simulink model "ss_robust_estimator_CT_real"  (R2022b)
settings: Solver=VariableStepAuto  StartTime=0.0  StopTime=10.0  FixedStep=Ts/20  RelTol=1e-3
undefined symbols (not defined in the file): degs2rpm, der, drv, gbox, mld, mot, rads2rpm, redObs, rpm2rads, sens, simul, ssNominal, ssRobust, Ts
settings Model: Creator=emanuelevitetta  LastModifiedBy=david

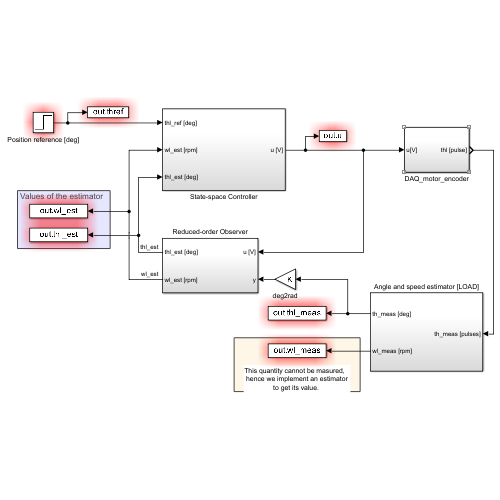
[thumbnail: Simulink's stored preview of the top-level diagram]
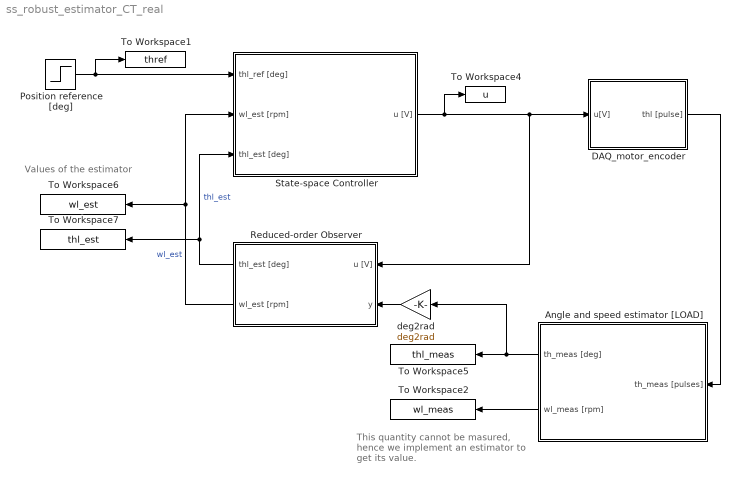
== system ss_robust_estimator_CT_real ==
  note: This quantity cannot be masured,
      | hence we implement an estimator
      | to get its value.
  note: Values of the estimator
  Angle and speed estimator [LOAD] : Subsystem
  DAQ_motor_encoder : Subsystem
  Position reference [deg] : Step  After=simul.stepdeg
  Reduced-order Observer : Subsystem
  State-space Controller : Subsystem
  To Workspace1 : ToWorkspace  VariableName=thref  SaveFormat=Structure With Time  SampleTime=Ts
  To Workspace2 : ToWorkspace  VariableName=wl_meas  SaveFormat=Structure With Time  SampleTime=Ts
  To Workspace4 : ToWorkspace  VariableName=u  SaveFormat=Structure With Time  SampleTime=Ts
  To Workspace5 : ToWorkspace  VariableName=thl_meas  SaveFormat=Structure With Time  SampleTime=Ts
  To Workspace6 : ToWorkspace  VariableName=wl_est  SaveFormat=Structure With Time  SampleTime=Ts
  To Workspace7 : ToWorkspace  VariableName=thl_est  SaveFormat=Structure With Time  SampleTime=Ts
  deg2rad : Gain  Gain=deg2rad
  wires:
  DAQ_motor_encoder/1(thl [pulse]) -> Angle and speed estimator [LOAD]/1(th_meas [pulses])
  Position reference [deg]/1 -> To Workspace1/1, State-space Controller/1(thl_ref [deg])
  Reduced-order Observer/2(wl_est [rpm]) -> To Workspace6/1, State-space Controller/2(wl_est [rpm])  "wl_est"
  State-space Controller/1(u [V]) -> To Workspace4/1, DAQ_motor_encoder/1(u[V]), Reduced-order Observer/1(u [V])
  Reduced-order Observer/1(thl_est [deg]) -> State-space Controller/3(thl_est [deg]), To Workspace7/1  "thl_est"
  deg2rad/1 -> Reduced-order Observer/2(y)
  Angle and speed estimator [LOAD]/1(th_meas [deg]) -> deg2rad/1, To Workspace5/1
  Angle and speed estimator [LOAD]/2(wl_meas [rpm]) -> To Workspace2/1

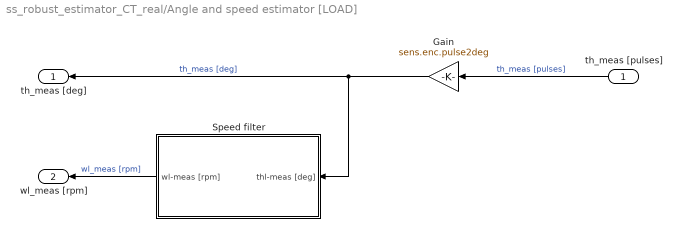
== system ss_robust_estimator_CT_real/Angle and speed estimator [LOAD] ==
  th_meas [pulses] : Inport
  Gain : Gain  Gain=sens.enc.pulse2deg
  Speed filter : Subsystem
  th_meas [deg] : Outport
  wl_meas [rpm] : Outport  Port=2
  wires:
  Speed filter/1(wl-meas [rpm]) -> wl_meas [rpm]/1  "wl_meas [rpm]"
  th_meas [pulses]/1 -> Gain/1  "th_meas [pulses]"
  Gain/1 -> Speed filter/1(thl-meas [deg]), th_meas [deg]/1  "th_meas [deg]"

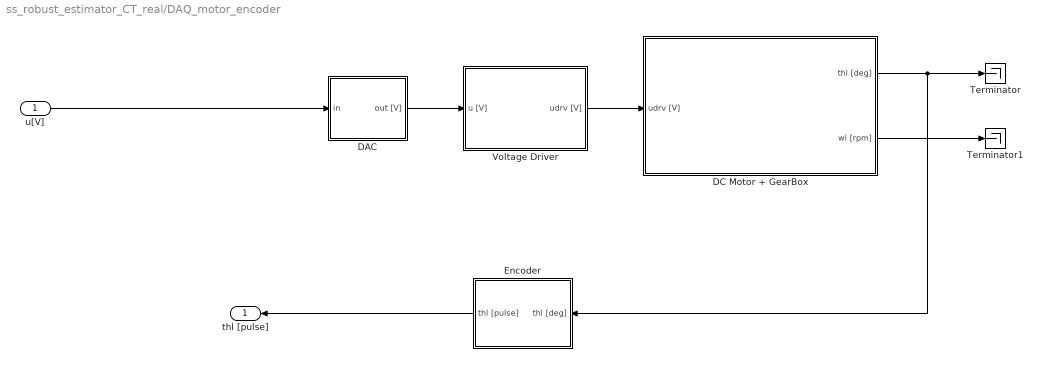
== system ss_robust_estimator_CT_real/DAQ_motor_encoder ==
  u[V] : Inport
  DAC : Subsystem
  DC Motor + GearBox : Subsystem
  Encoder : Subsystem
  Terminator : Terminator
  Terminator1 : Terminator
  Voltage Driver : Subsystem
  thl [pulse] : Outport
  wires:
  DC Motor + GearBox/1(thl [deg]) -> Encoder/1(thl [deg]), Terminator/1
  DC Motor + GearBox/2(wl [rpm]) -> Terminator1/1
  Voltage Driver/1(udrv [V]) -> DC Motor + GearBox/1(udrv [V])
  u[V]/1 -> DAC/1(in)
  DAC/1(out [V]) -> Voltage Driver/1(u [V])
  Encoder/1(thl [pulse]) -> thl [pulse]/1

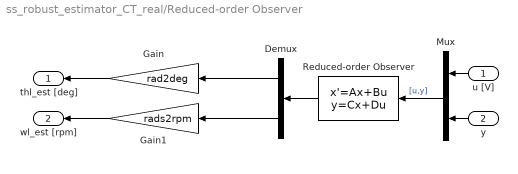
== system ss_robust_estimator_CT_real/Reduced-order Observer ==
  u [V] : Inport
  y : Inport  Port=2
  Demux : Demux  Outputs=2
  Gain : Gain  Gain=rad2deg
  Gain1 : Gain  Gain=rads2rpm
  Mux : Mux  Inputs=2
  Reduced-order Observer : StateSpace  A=redObs.A0  B=redObs.B0  C=redObs.C0  D=redObs.D0  InitialCondition=0  ParameterTunability=Unconstrained
  thl_est [deg] : Outport
  wl_est [rpm] : Outport  Port=2
  wires:
  Demux/1 -> Gain/1
  Mux/1 -> Reduced-order Observer/1  "[u,y]"
  Demux/2 -> Gain1/1
  y/1 -> Mux/2
  u [V]/1 -> Mux/1
  Reduced-order Observer/1 -> Demux/1
  Gain/1 -> thl_est [deg]/1
  Gain1/1 -> wl_est [rpm]/1

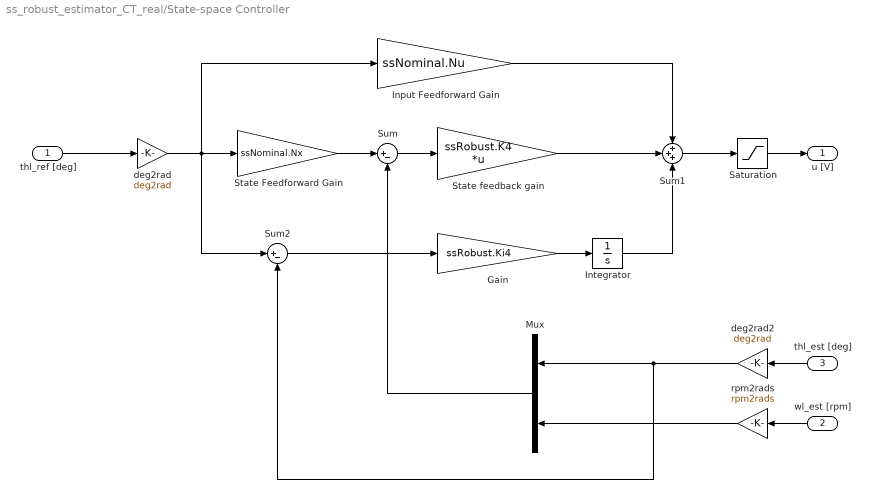
== system ss_robust_estimator_CT_real/State-space Controller ==
  thl_ref [deg] : Inport
  wl_est [rpm] : Inport  Port=2
  thl_est [deg] : Inport  Port=3
  Gain : Gain  Gain=ssRobust.Ki4
  Input Feedforward Gain : Gain  Gain=ssNominal.Nu
  Integrator : Integrator
  Mux : Mux  Inputs=2
  Saturation : Saturate  UpperLimit=10  LowerLimit=-10
  State Feedforward Gain : Gain  Gain=ssNominal.Nx
  State feedback gain : Gain  Gain=ssRobust.K4  Multiplication=Matrix(K*u)
  Sum : Sum  Inputs=|+-
  Sum1 : Sum  Inputs=+++
  Sum2 : Sum  Inputs=|+-
  deg2rad : Gain  Gain=deg2rad
  deg2rad2 : Gain  Gain=deg2rad
  rpm2rads : Gain  Gain=rpm2rads
  u [V] : Outport
  wires:
  thl_est [deg]/1 -> deg2rad2/1
  wl_est [rpm]/1 -> rpm2rads/1
  Mux/1 -> Sum/2
  thl_ref [deg]/1 -> deg2rad/1
  deg2rad/1 -> Sum2/1, State Feedforward Gain/1, Input Feedforward Gain/1
  State Feedforward Gain/1 -> Sum/1
  Sum/1 -> State feedback gain/1
  State feedback gain/1 -> Sum1/2
  Sum1/1 -> Saturation/1
  Input Feedforward Gain/1 -> Sum1/1
  Gain/1 -> Integrator/1
  Integrator/1 -> Sum1/3
  Sum2/1 -> Gain/1
  deg2rad2/1 -> Mux/1, Sum2/2
  rpm2rads/1 -> Mux/2
  Saturation/1 -> u [V]/1

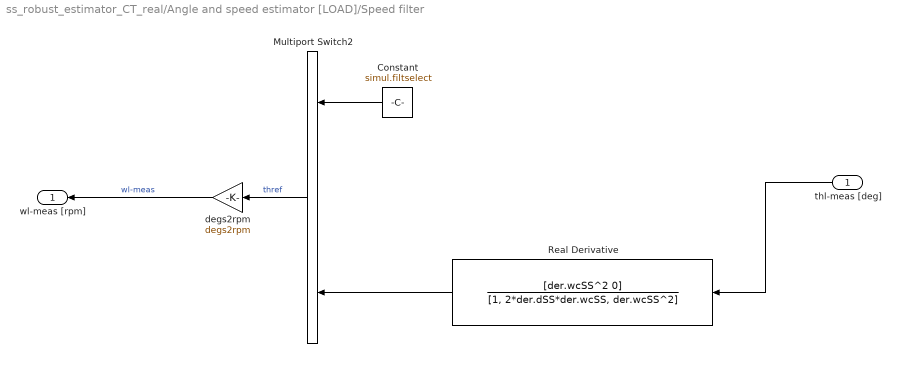
== system ss_robust_estimator_CT_real/Angle and speed estimator [LOAD]/Speed filter ==
  thl-meas [deg] : Inport
  Constant : Constant  Value=simul.filtselect
  Multiport Switch2 : MultiPortSwitch  Inputs=2  SaturateOnIntegerOverflow=off  InputSameDT=off
  Real Derivative : TransferFcn  Numerator=[der.wcSS^2 0]  Denominator=[1, 2*der.dSS*der.wcSS, der.wcSS^2]
  degs2rpm : Gain  Gain=degs2rpm
  wl-meas [rpm] : Outport
  wires:
  degs2rpm/1 -> wl-meas [rpm]/1  "wl-meas"
  Real Derivative/1 -> Multiport Switch2/3
  Multiport Switch2/1 -> degs2rpm/1  "thref"
  Constant/1 -> Multiport Switch2/1
  thl-meas [deg]/1 -> Real Derivative/1

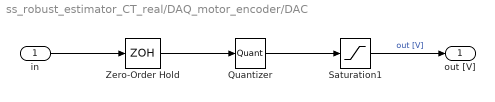
== system ss_robust_estimator_CT_real/DAQ_motor_encoder/DAC ==
  in : Inport
  Quantizer : Quantizer  QuantizationInterval=daq.dac.q
  Saturation1 : Saturate  UpperLimit=10  LowerLimit=-10
  Zero-Order Hold : ZeroOrderHold  SampleTime=0.001
  out [V] : Outport
  wires:
  Saturation1/1 -> out [V]/1  "out [V]"
  in/1 -> Zero-Order Hold/1
  Zero-Order Hold/1 -> Quantizer/1
  Quantizer/1 -> Saturation1/1

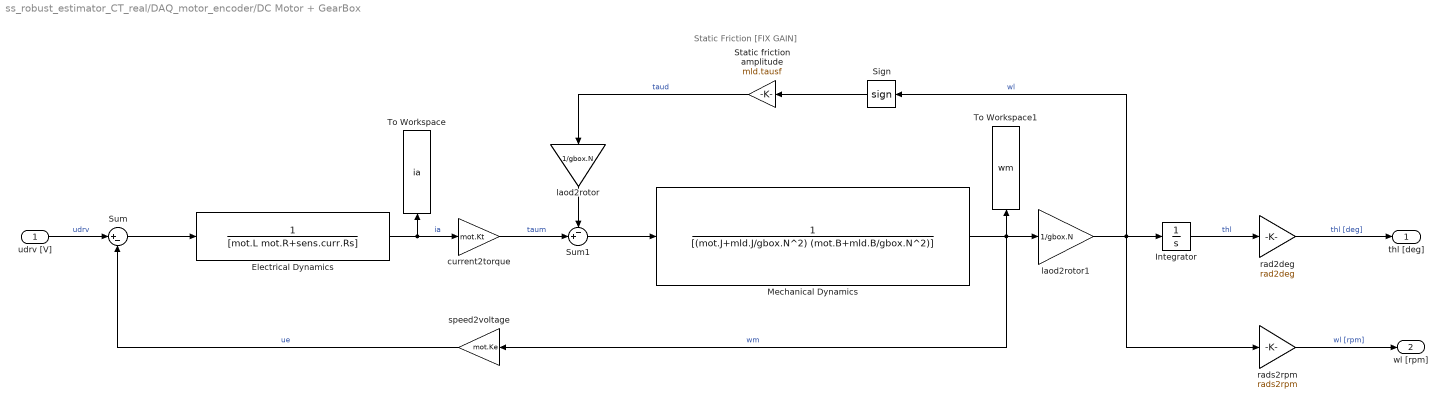
== system ss_robust_estimator_CT_real/DAQ_motor_encoder/DC Motor + GearBox ==
  note: Static Friction [FIX GAIN]
  udrv [V] : Inport
  Electrical Dynamics : TransferFcn  Denominator=[mot.L mot.R+sens.curr.Rs]
  Integrator : Integrator
  Mechanical Dynamics : TransferFcn  Denominator=[(mot.J+mld.J/gbox.N^2) (mot.B+mld.B/gbox.N^2)]
  Sign : Signum  ZeroCross=off
  Static friction amplitude : Gain  Gain=mld.tausf
  Sum : Sum  Inputs=|+-
  Sum1 : Sum  Inputs=-+|
  To Workspace : ToWorkspace  VariableName=ia  SaveFormat=Timeseries  SampleTime=-1
  To Workspace1 : ToWorkspace  VariableName=wm  SaveFormat=Timeseries  SampleTime=-1
  current2torque : Gain  Gain=mot.Kt
  laod2rotor : Gain  Gain=1/gbox.N
  laod2rotor1 : Gain  Gain=1/gbox.N
  rad2deg : Gain  Gain=rad2deg
  rads2rpm : Gain  Gain=rads2rpm
  speed2voltage : Gain  Gain=mot.Ke
  thl [deg] : Outport
  wl [rpm] : Outport  Port=2
  wires:
  rads2rpm/1 -> wl [rpm]/1  "wl [rpm]"
  Sign/1 -> Static friction amplitude/1
  Electrical Dynamics/1 -> To Workspace/1, current2torque/1  "ia"
  Sum1/1 -> Mechanical Dynamics/1
  laod2rotor1/1 -> rads2rpm/1, Sign/1, Integrator/1  "wl"
  rad2deg/1 -> thl [deg]/1  "thl [deg]"
  laod2rotor/1 -> Sum1/1
  udrv [V]/1 -> Sum/1  "udrv"
  current2torque/1 -> Sum1/2  "taum"
  Static friction amplitude/1 -> laod2rotor/1  "taud"
  speed2voltage/1 -> Sum/2  "ue"
  Integrator/1 -> rad2deg/1  "thl"
  Sum/1 -> Electrical Dynamics/1
  Mechanical Dynamics/1 -> laod2rotor1/1, To Workspace1/1, speed2voltage/1  "wm"

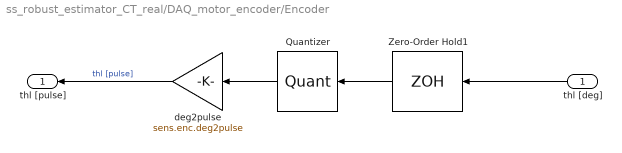
== system ss_robust_estimator_CT_real/DAQ_motor_encoder/Encoder ==
  thl [deg] : Inport
  Quantizer : Quantizer  QuantizationInterval=sens.enc.pulse2deg
  Zero-Order Hold1 : ZeroOrderHold  SampleTime=0.001
  deg2pulse : Gain  Gain=sens.enc.deg2pulse
  thl [pulse] : Outport
  wires:
  thl [deg]/1 -> Zero-Order Hold1/1
  Zero-Order Hold1/1 -> Quantizer/1
  deg2pulse/1 -> thl [pulse]/1  "thl [pulse]"
  Quantizer/1 -> deg2pulse/1

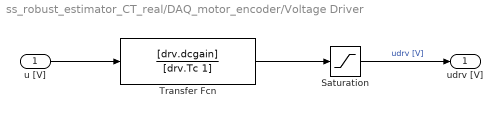
== system ss_robust_estimator_CT_real/DAQ_motor_encoder/Voltage Driver ==
  u [V] : Inport
  Saturation : Saturate  UpperLimit=12  LowerLimit=-12
  Transfer Fcn : TransferFcn  Numerator=[drv.dcgain]  Denominator=[drv.Tc 1]
  udrv [V] : Outport
  wires:
  Saturation/1 -> udrv [V]/1  "udrv [V]"
  u [V]/1 -> Transfer Fcn/1
  Transfer Fcn/1 -> Saturation/1
